simulink model "QuadcopterSimPartD"  (R2025a)
settings: Solver=ode45  StartTime=0.0  StopTime=500  MaxStep=1  RelTol=1e-3  EnableMultiTasking=on
values from neighbouring files (symbols this model uses):
  g = 9.81    [QuadcopterPlots.m]
  h0 = 1    [QuadcopterPlots.m]
  hdot0 = 0    [QuadcopterPlots.m]
  kT = m*g/4/u_average_per_motor    [QuadcopterPlots.m]
  m = 65e-3    (= 0.065)    [QuadcopterPlots.m]
  umax = 500    [QuadcopterPlots.m]
settings Model: Creator=pjseiler  LastModifiedBy=Alex_
settings SolverCC: AlgebraicLoopSolver=TrustRegion
settings DataIOCC: LimitDataPoints=on  SaveFormat=Array  SignalLoggingSaveFormat=ModelDataLogs  ReturnWorkspaceOutputs=off
settings OptimizationCC: ExpressionDepthLimit=2147483647.0  LifeSpan=inf
settings DebuggingCC: UnderspecifiedInitializationDetection=Classic  MergeDetectMultiDrivingBlocksExec=none  SolverPrmCheckMsg=warning  FcnCallInpInsideContextMsg=warning  UnconnectedInputMsg=warning  UnconnectedOutputMsg=warning  UnconnectedLineMsg=warning  StateNameClashWarn=warning  SFUnexpectedBacktrackingDiag=warning  SFNoUnconditionalDefaultTransitionDiag=warning  ArithmeticOperatorsInVariantConditions=warning
settings HardwareCC: ProdBitPerPointer=32.0  ProdBitPerSizeT=32.0  ProdBitPerPtrDiffT=32.0  ProdLargestAtomicFloat=None  ProdIntDivRoundTo=Undefined  ProdEndianess=Unspecified  ProdWordSize=32.0  ProdHWDeviceType=32-bit Generic
settings ModelReferenceCC: EnableRefExpFcnMdlSchedulingChecks=on  PropagateSignalLabelsOutOfModel=off
settings SFSimCC: SimUseLocalCustomCode=off  CustomCodeUndefinedFunction=UseInterfaceOnly
settings RTWCC: RTWUseLocalCustomCode=off  GPUComputeCapability=3.5
settings CodeAppCC: StateflowObjectComments=on
settings GRTTargetCC: TargetLangStandard=C89/C90 (ANSI)  CombineOutputUpdateFcns=off  GRTInterface=on
settings ConfigComp: CovMetricSettings=dw  CovSaveCumulativeToWorkspaceVar=on  CovSaveSingleToWorkspaceVar=on  CovExternalEMLEnable=off

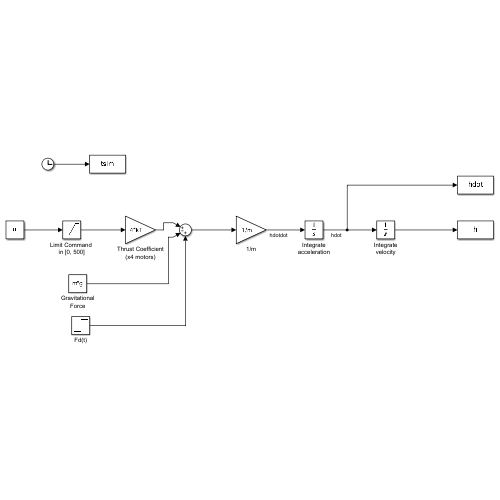
[thumbnail: Simulink's stored preview of the top-level diagram]
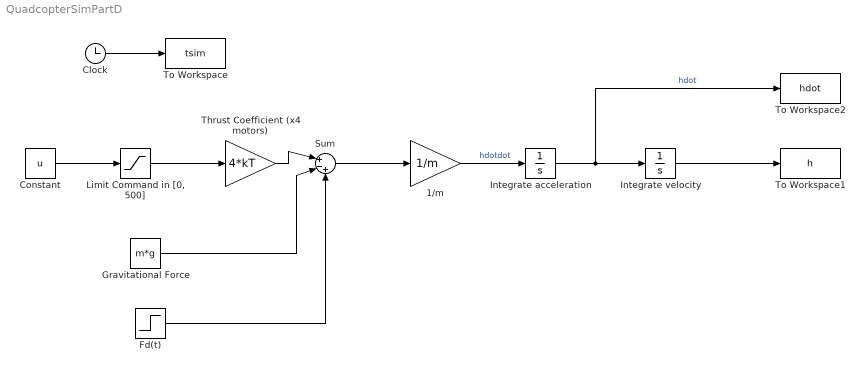
== system QuadcopterSimPartD ==
  1/m : Gain  Gain=1/m
  Clock : Clock
  Constant : Constant  Value=u
  Fd(t) : Step  Time=5  After=0.05  SampleTime=0
  Gravitational Force : Constant  Value=m*g
  Integrate acceleration : Integrator  InitialCondition=hdot0
  Integrate velocity : Integrator  InitialCondition=h0
  "Limit Command in [0, 500]" : Saturate  UpperLimit=umax  LowerLimit=0
  Sum : Sum  Inputs=|+-+
  Thrust Coefficient (x4 motors) : Gain  Gain=4*kT
  To Workspace : ToWorkspace  VariableName=tsim  SampleTime=-1
  To Workspace1 : ToWorkspace  VariableName=h  SampleTime=-1
  To Workspace2 : ToWorkspace  VariableName=hdot  SampleTime=-1
  wires:
  Clock/1 -> To Workspace/1
  Sum/1 -> 1/m/1
  Thrust Coefficient (x4 motors)/1 -> Sum/1
  1/m/1 -> Integrate acceleration/1  "hdotdot"
  Constant/1 -> "Limit Command in [0, 500]"/1
  Integrate velocity/1 -> To Workspace1/1
  Integrate acceleration/1 -> To Workspace2/1, Integrate velocity/1  "hdot"
  Gravitational Force/1 -> Sum/2
  "Limit Command in [0, 500]"/1 -> Thrust Coefficient (x4 motors)/1
  Fd(t)/1 -> Sum/3
